simulink model "Observabilidad_simu"  (R2021a)
settings: Solver=VariableStepAuto  StartTime=0.0  StopTime=10.0  RelTol=1e-3
values from neighbouring files (symbols this model uses):
  A = [-2 -1; 0 -4]    [Control_Integral.m]    (also in Controlabilidad.m = P.a; Ejemplo_filminas.m = SS.A; Ejercicio_Inestable.m = [100, 0; 160, 200]; Ejercicio_Valvulas.m = double(A))
  B = [1; 0]    [Control_Integral.m]    (also in Controlabilidad.m = P.b; Ejemplo_filminas.m = SS.B; Ejercicio_Inestable.m = [70; 160]; Ejercicio_Valvulas.m = double(B))
  C = [1 1]    [Control_Integral.m]    (also in Controlabilidad.m = P.c; Ejemplo_filminas.m = SS.C; Ejercicio_Inestable.m = [1, 1]; Ejercicio_Valvulas.m = double(C))
  L = zpk(ceros, polos, ganancia)    [Ejemplo_filminas.m]    (also in Ejercicio_Inestable.m = inv(Wo) * Wom * [l1 - a1; l2 - a2]; Observabilidad.m = [18; 99]; realimentacion_ee.m = [18; 99])
settings Model: Creator=Santiago  LastModifiedBy=Santiago

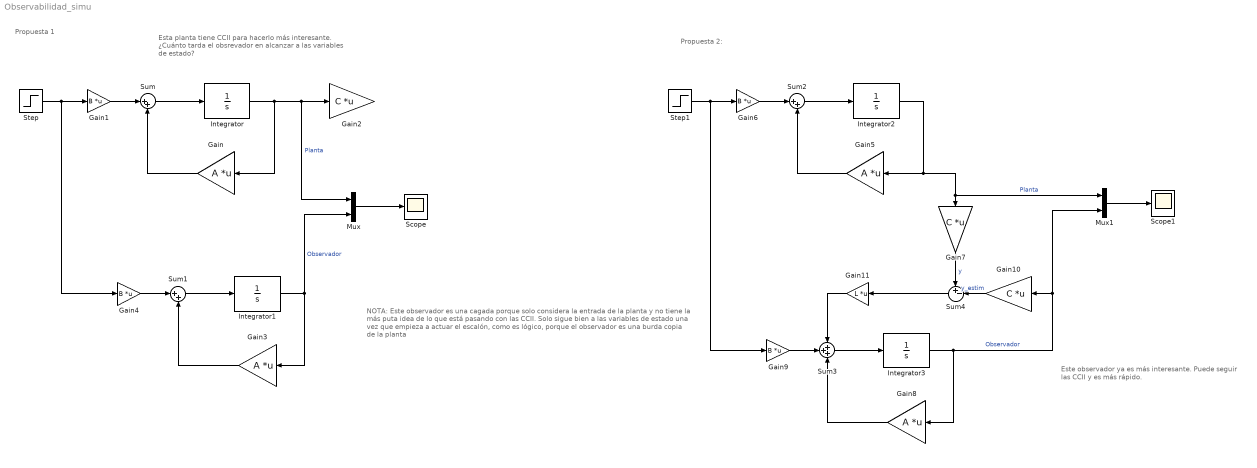
== system Observabilidad_simu ==
  note: Este observador ya es más interesante. Puede seguir las CCII y es más rápido.
  note: Propuesta 1
  note: Propuesta 2:
  note: NOTA: Este observador es una cagada porque solo considera la entrada de la planta y no tiene la más puta idea de lo que está pasando con las CCII. Solo sigue bien a las variables de estado una vez que empieza a actuar el escalón, como es lógico, porque el observador es una burda copia de la planta
  note: Esta planta tiene CCII para hacerlo más interesante. ¿Cuánto tarda el obsrevador en alcanzar a las variables de estado?
  Gain{,3,5,8} (4 alike) : Gain  Gain=A  Multiplication=Matrix(K*u) (u vector)
  Gain{1,4,6,9} (4 alike) : Gain  Gain=B  Multiplication=Matrix(K*u)
  Gain10 : Gain  Gain=C  Multiplication=Matrix(K*u) (u vector)
  Gain11 : Gain  Gain=L  Multiplication=Matrix(K*u)
  Gain2 : Gain  Gain=C  Multiplication=Matrix(K*u) (u vector)
  Gain7 : Gain  Gain=C  Multiplication=Matrix(K*u) (u vector)
  Integrator : Integrator  InitialCondition=[10 10]
  Integrator1 : Integrator
  Integrator2 : Integrator  InitialCondition=[10 10]
  Integrator3 : Integrator
  Mux : Mux  Inputs=2
  Mux1 : Mux  Inputs=2
  Scope : Scope
  Scope1 : Scope
  Step : Step  Time=5  After=10  SampleTime=0
  Step1 : Step  Time=5  After=10  SampleTime=0
  Sum : Sum  Inputs=|++
  Sum1 : Sum  Inputs=|++
  Sum2 : Sum  Inputs=|++
  Sum3 : Sum  Inputs=+++
  Sum4 : Sum  Inputs=+-|
  wires:
  Integrator/1 -> Mux/1, Gain2/1, Gain/1  "Planta"
  Sum/1 -> Integrator/1
  Gain/1 -> Sum/2
  Gain1/1 -> Sum/1
  Sum1/1 -> Integrator1/1
  Gain4/1 -> Sum1/1
  Step/1 -> Gain4/1, Gain1/1
  Gain3/1 -> Sum1/2
  Integrator1/1 -> Mux/2, Gain3/1  "Observador"
  Mux/1 -> Scope/1
  Integrator3/1 -> Mux1/2, Gain10/1, Gain8/1  "Observador"
  Integrator2/1 -> Gain7/1, Mux1/1, Gain5/1  "Planta"
  Sum2/1 -> Integrator2/1
  Gain6/1 -> Sum2/1
  Mux1/1 -> Scope1/1
  Step1/1 -> Gain9/1, Gain6/1
  Gain5/1 -> Sum2/2
  Sum3/1 -> Integrator3/1
  Gain7/1 -> Sum4/1  "y"
  Gain10/1 -> Sum4/2  "y_estim"
  Sum4/1 -> Gain11/1
  Gain8/1 -> Sum3/3
  Gain9/1 -> Sum3/2
  Gain11/1 -> Sum3/1
